simulink model "full_scale_car"  (R2024b)
settings: Solver=ode23t  StartTime=0.0  StopTime=25  MaxStep=1e-4  MinStep=1e-7  RelTol=1e-3
libraries: spsGroundLib x8, spsVoltageMeasurementLib x4, nesl_utility x4, spsControlledCurrentSourceLib x3, spsCurrentMeasurementLib x3, spsDCVoltageSourceLib x2, sdl_lib x2, spsSeriesRLCBranchLib x2, spsDCMachineLib x1, spsControlledVoltageSourceLib x1, fl_lib x1, simulink x1
settings Model: Creator=adamo  LastModifiedBy=adamo
settings SolverCC: ShapePreserveControl=EnableAll

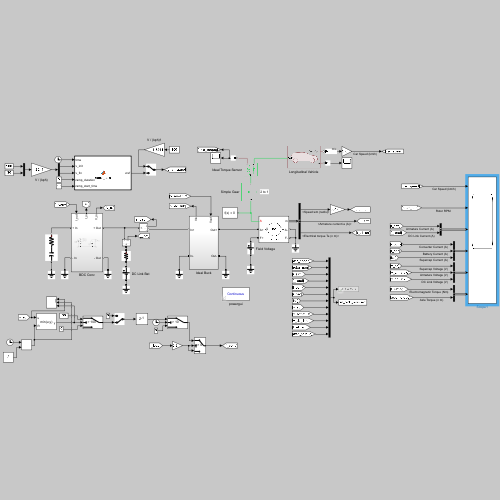
[thumbnail: Simulink's stored preview of the top-level diagram]
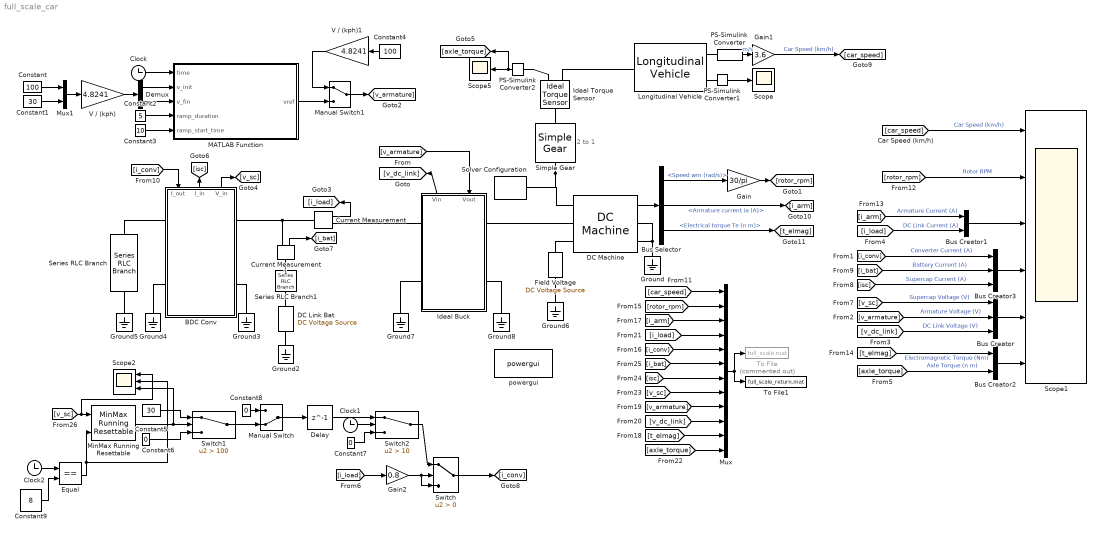
== system full_scale_car ==
  note: 2 to 1
  BDC Conv : Subsystem
      settings: PortSchema="{\"entries\":[{\"content\":{\"sides\":[{\"content\":{\"connectorIds\":[\"LConn1\",\"LConn2\"]},\"type\":\"ConnectorPlacement.EquallySpacedRectSide\",\"uuid\":\"9f090672-6a88-4e94-aaf3-d933b370ecea\"},{\"content\":{\"connectorIds\":[\"RConn1\",\"RConn2\"],\"side\":\"RIGHT\"},\"type\":\"ConnectorPlacement.EquallySpacedRectSide\",\"uuid\":\"4ec5d7b0-9e11-491f-a704-2c93c36a28cb\"},{\"content\":{\"connectorIds\":[\"In1\",\"Out1\",\"Out2\"],\"side\":\"TOP\"},\"type\":\"ConnectorPlacement.EquallySpacedRectSide\",\"uuid\":\"1397e6b8-a84b-4f43-abb0-36c2f8d57e37\"}]},\"type\":\"ConnectorPlacement.EquallySpacedConnector\",\"uuid\":\"02ba4b3a-9b7c-4d0b-ba36-63e783e5597b\"}],\"packageUris\":[\"http://schema.mathworks.com/mf0/Connector/R2020b\"],\"version\":\"1.0\"}"
  Bus Creator : BusCreator  Inputs=3
  Bus Creator1 : BusCreator  Inputs=2
  Bus Creator2 : BusCreator  Inputs=2
  Bus Creator3 : BusCreator  Inputs=3
  Bus Selector : BusSelector  OutputSignals=Speed wm (rad/s),Armature current ia (A),Electrical torque Te (n m)
  Clock : Clock
  Clock1 : Clock
  Clock2 : Clock
  Constant : Constant  Value=100
  Constant1 : Constant  Value=30
  Constant2 : Constant  Value=5
  Constant3 : Constant  Value=10
  Constant4 : Constant  Value=100
  Constant5 : Constant  Value=30
  Constant6 : Constant  Value=0
  Constant7 : Constant  Value=0
  Constant8 : Constant  Value=0
  Constant9 : Constant  Value=8
  Current Measurement : spsCurrentMeasurementLib/Current Measurement  PhasorSimulation=off  OutputType=Complex  PSBequivalent=0
  Current Measurement1 : spsCurrentMeasurementLib/Current Measurement  PhasorSimulation=off  OutputType=Complex  PSBequivalent=0
  DC Link Bat : spsDCVoltageSourceLib/DC Voltage Source  Amplitude=500  Measurements=None
  DC Machine : spsDCMachineLib/DC Machine  PresetModel=23: 250HP 500V 1750RPM Field:300V  MechanicalLoad=Mechanical rotational port  FieldType=Wound  ShowDetailedParameters=on  MeasurementBus=off  RLa=[0.06727 0.001882]  RLf=[30.72 3.166]  Laf=0.2641  MachineConstant=Torque constant (N.m/A)  Ke=1.8  Kt=1.8  J=1.019  Bm=0.02516  Tf=26.46  w0=190  Ifinit=9.76562499959051  TsPowergui=0  TsBlock=-1
  Delay : Delay  DelayLength=1
  Demux : Demux  Outputs=2
  Equal : RelationalOperator  Operator===  OutDataTypeStr=boolean  RndMeth=Simplest  InputSameDT=off
  Field Voltage : spsDCVoltageSourceLib/DC Voltage Source  Amplitude=300  Measurements=None
  Gain : Gain  Gain=30/pi
  Gain1 : Gain  Gain=3.6
  Gain2 : Gain  Gain=0.8
  Ground{,2..8} (8 alike) : spsGroundLib/Ground  LConnTagsString=a
  Ideal Buck : Subsystem
      settings: PortSchema="{\"entries\":[{\"content\":{\"sides\":[{\"content\":{\"connectorIds\":[\"LConn1\",\"LConn2\"]},\"type\":\"ConnectorPlacement.EquallySpacedRectSide\",\"uuid\":\"35f6ef1c-d887-4ecf-80f2-2c39dcd17f78\"},{\"content\":{\"connectorIds\":[\"RConn1\",\"RConn2\"],\"side\":\"RIGHT\"},\"type\":\"ConnectorPlacement.EquallySpacedRectSide\",\"uuid\":\"8a3f3d43-a013-4f94-8838-6f4ac1397b41\"},{\"content\":{\"connectorIds\":[\"Out1\",\"In1\"],\"side\":\"TOP\"},\"type\":\"ConnectorPlacement.EquallySpacedRectSide\",\"uuid\":\"6e5b1b24-962b-4715-9a1c-61b4175c500b\"}]},\"type\":\"ConnectorPlacement.EquallySpacedConnector\",\"uuid\":\"9f7927fc-518e-4b31-bc3b-cadb6b312eb4\"}],\"packageUris\":[\"http://schema.mathworks.com/mf0/Connector/R2020b\"],\"version\":\"1.0\"}"
  Ideal Torque Sensor : fl_lib/Mechanical/Mechanical Sensors/Ideal Torque Sensor
  Longitudinal Vehicle : sdl_lib/Tires & Vehicles/Longitudinal Vehicle  vehParamType=sdl.enum.VehicleParameterizationType.Regular  M_vehicle=2000 kg  R_tireroll=0.3 m  C_tireroll=0.0136  C_airdrag=0.4  A_front=2.3 m^2  A_rl=120 N  B_rl=1.8 N*s/m  C_rl=0.389 N*s^2/m^2  g=9.81 m/s^2  V_1=0.3 m/s  w_1=0.01 rad/s  ShowBrakeIn=false  ShowSlopeIn=false  SlopeInputType=sdl.enum.VehicleLongitudinalRoadSlopeInputType.GradePercent  ShowWindIn=false  ShowGOut=true  air_density=1.184 kg/m^3  V_x_specify=on  V_x_priority=High  V_x=100 kph  V_x_nominal_specify=on  V_x_nominal_value=100  V_x_nominal_unit=kph  trq_specify=off  trq_priority=None  trq=0 N*m  trq_nominal_specify=on  trq_nominal_value=150  trq_nominal_unit=N*m  w_specify=off  w_priority=None  w=0 rad/s  w_nominal_specify=on  w_nominal_value=190/3  w_nominal_unit=rad/s
      settings: InternalSimscapePortConfiguration="{\"Bottom\":[],\"Left\":[{\"id\":\"Axle\",\"label\":\"Axle\",\"type\":\"foundation.mechanical.rotational.rotational\"}],\"Right\":[{\"id\":\"v_out\",\"label\":\"VehSpd\",\"type\":\"output\"},{\"id\":\"G_out\",\"label\":\"G\",\"type\":\"output\"}],\"Top\":[]}"
  MATLAB Function : MATLAB Function  TreatAsAtomicUnit=on
  Manual Switch : ManualSwitch  CurrentSetting=0
  Manual Switch1 : ManualSwitch
  MinMax Running Resettable : simulink/Math Operations/MinMax Running Resettable  Function=min  vinit=200
  Mux : Mux  Inputs=12
  Mux1 : Mux  Inputs=2
  PS-Simulink Converter : nesl_utility/PS-Simulink Converter  PhysicalDomain=network_engine_domain  SubClassName=ps_output  LeftPortType=input  RightPortType=output  PseudoPeriodic=off  Frequencies=[]  VectorFormat=inherit  Unit=inherit  AffineConversion=off
  PS-Simulink Converter1 : nesl_utility/PS-Simulink Converter  PhysicalDomain=network_engine_domain  SubClassName=ps_output  LeftPortType=input  RightPortType=output  PseudoPeriodic=off  Frequencies=[]  VectorFormat=inherit  Unit=inherit  AffineConversion=off
  PS-Simulink Converter2 : nesl_utility/PS-Simulink Converter  PhysicalDomain=network_engine_domain  SubClassName=ps_output  LeftPortType=input  RightPortType=output  PseudoPeriodic=off  Frequencies=[]  VectorFormat=inherit  Unit=inherit  AffineConversion=off
  Scope : Scope
  Scope1 : Scope  NumInputPorts=6
  Scope2 : Scope  NumInputPorts=3
  Scope5 : Scope
  Series RLC Branch : spsSeriesRLCBranchLib/Series RLC Branch  LConnTagsString=__new0  RConnTagsString=__new0  BranchType=RC  Resistance=10e-3  Inductance=1e-3  SetiL0=off  InitialCurrent=0  Capacitance=20  Setx0=on  InitialVoltage=150  Measurements=None
  Series RLC Branch1 : spsSeriesRLCBranchLib/Series RLC Branch  LConnTagsString=__new0  RConnTagsString=__new0  BranchType=R  Resistance=10e-3  Inductance=1e-3  SetiL0=off  InitialCurrent=0  Capacitance=10  Setx0=on  InitialVoltage=250/4  Measurements=None
  Simple Gear : sdl_lib/Gears/Simple Gear  ratio=2  rotation_direction=sdl.enum.shaftOutputDirection.same  friction_model=sdl.enum.gear_efficiencies_load.off  T_noload=0.1 N*m  T_nom=5 N*m  efficiency_nom=0.8  efficiency=0.8  temperature_TLU=[280, 300, 320] K  load_TLU=[1, 5, 10] N*m  efficiency_TLU=[.95, .9, .85]  efficiency_TLU2=[.85, .8, .75; .95, .9, .85; .85, .8, .7]  w_thr=0.01 rad/s  pwr_thr=0.001 W  enable_backlash=false  hardstop_model=simscape.enum.hardstop.smooth  backlash_distance=1e-3 mm  r_base=0.1 m  transition=1e-4 mm  backlash_stiffness=1e6 N/m  backlash_damping=1e3 N*s/m  coeff_rest=0.7  v_tol=0.001 m/s  f_tol=0.001 N  mu_visc=[0, 0] N*m*s/rad  thermal_mass=50 J/K  temperature_specify=off  temperature_priority=High  temperature=300 K  temperature_nominal_specify=off  temperature_nominal_value=1  temperature_nominal_unit=K  x_backlash_specify=off  x_backlash_priority=None  x_backlash=0 mm  x_backlash_nominal_specify=off  x_backlash_nominal_value=1  x_backlash_nominal_unit=mm  f_hardstop_specify=off  f_hardstop_priority=None  f_hardstop=0 N  f_hardstop_nominal_specify=off  f_hardstop_nominal_value=1  f_hardstop_nominal_unit=N  v_backlash_specify=off  v_backlash_priority=None  v_backlash=0 m/s  v_backlash_nominal_specify=off  v_backlash_nominal_value=1  v_backlash_nominal_unit=m/s
  Solver Configuration : nesl_utility/Solver Configuration  PhysicalDomain=network_engine_domain  SubClassName=solver  LeftPortType=input  RightPortType=generic  Tones=[]  Harmonics=[]  SimulateNoise=off  Profile=off  UseLocalSampling=off  EnableSwitchedLinearOptims=on  FrequencyDomain=off  UseCCode=off  RelTol=0.001  AbsTol=0.001  MinStep=1e-09  ToWorkspace=off  RevertToSquareIcSolve=off  NumHomotopyIterations=100  PhasorMode=off  PhasorModeNumHarmonics=1  ConsistencySolver=NEWTON_XTOL_AFTER_FTOL  IndexReductionMethod=DerivativeReplacement  DoDC=off  ResidualTolerance=1e-09  ConsistencyTolSource=GLOBAL  ConsistencyAbsTol=0.001  ConsistencyRelTol=0.001  ConsistencyTolFactor=0.001  UseLocalSolver=off  LocalSolverChoice=NE_BACKWARD_EULER_ADVANCER  ResolveIndetEquations=on  FunctionEvalNumThread=1  LocalSolverSampleTime=0.001  DoFixedCost=off  MaxNonlinIter=3  MaxModeIter=2  ComputeImpulses=off  ImpulseIterations=2  LinearAlgebra=auto  LinearAlgebraNumThread=0  EquationFormulation=NE_TIME_EF  DelaysMemoryBudget=1024  AutomaticFiltering=on  FilteringTimeConstant=0.001  PartitionStorageMethod=AS_NEEDED  PartitionMemoryBudget=1024  PartitionMethod=ROBUST  MultibodyUseLocalSolver=off  MultibodyLocalSolverChoice=ODE1  MultibodyLocalSolverSampleTime=0.001
  Switch : Switch  Criteria=u2 > Threshold  SaturateOnIntegerOverflow=off  InputSameDT=off
  Switch1 : Switch  Criteria=u2 > Threshold  Threshold=100  SaturateOnIntegerOverflow=off  InputSameDT=off
  Switch2 : Switch  Criteria=u2 > Threshold  Threshold=10  SaturateOnIntegerOverflow=off  InputSameDT=off
  To File : ToFile  Commented=on  Filename=full_scale.mat  MatrixName=fs_ans
  To File1 : ToFile  Filename=full_scale_return.mat  MatrixName=fs_ans
  V / (kph) : Gain  Gain=4.8241
  V / (kph)1 : Gain  Gain=4.8241
  powergui : spspowerguiLib/powergui  Priority=1  SimulationMode=Continuous  SampleTime=50e-6  frequency=60  Iterations=50  frequencyindice=0  Pbase=100e6  ErrMax=1e-4  UnitsV=kV  UnitsW=MW  buscounter=0  FunctionMessages=off  echomessages=off  EnableUseOfTLC=off  CurrentSourceSwitches=off  DisableSnubberDevices=on  DisableRonSwitches=on  DisableVfSwitches=on  DisplayEquations=off  AutomaticDiscreteSolvers=off  SolverType=Tustin/Backward Euler (TBE)  Interpol=off  ExternalGateDelay=off  methode=off  Ts=100  x0status=blocks  SPID=on  SwTol=0  HookPort=off  NonlinearTolerance=1e-4  nMaxIteration=100  ContinueOnMaxIteration=off  RestoreLinks=warning  ResistiveCurrentMeasurement=off  Frange=[0:2:500]  Ylog=off  Xlog=on  ShowGrid=off  save=off  variable=ZData  structure=0  ZoomFFT=off  StartTime=0.0  cycles=1  DisplayStyle=1  fundamental=60  FreqAxis=off  MaxFrequency=1000  frequencyindicesteady=1  RmsSteady=1  display=off
  wires:
  [axle_torque] -> Bus Creator2/2  "Axle Torque (n m)"
  Gain1/1 -> [car_speed]  "Car Speed (km/h)"
  Bus Selector/2 -> [i_arm]  "<Armature current ia (A)>"
  Bus Creator/1 -> Scope1/5
  Bus Selector/1 -> Gain/1  "<Speed wm (rad/s)>"
  Gain/1 -> [rotor_rpm]
  [t_elmag] -> Bus Creator2/1  "Electromagnetic Torque (Nm)"
  Bus Creator2/1 -> Scope1/6
  Bus Creator1/1 -> Scope1/3
  DC Machine/1 -> Bus Selector/1
  [i_load] -> Bus Creator1/2  "DC Link Current (A)"
  PS-Simulink Converter2/1 -> [axle_torque], Scope5/1
  PS-Simulink Converter/1 -> Gain1/1  "m/s"
  [v_armature] -> Bus Creator/2  "Armature Voltage (V)"
  [v_dc_link] -> Bus Creator/3  "DC Link Voltage (V)"
  Current Measurement/1 -> [i_load]
  MATLAB Function/1(vref) -> Manual Switch1/2
  [v_armature] -> Ideal Buck/1(Vout)
  Ideal Buck/1(Vin) -> [v_dc_link]
  Clock/1 -> MATLAB Function/1(time)
  Constant2/1 -> MATLAB Function/4(ramp_duration)
  Constant3/1 -> MATLAB Function/5(ramp_start_time)
  [v_sc] -> Bus Creator/1  "Supercap Voltage (V)"
  [isc] -> Bus Creator3/3  "Supercap Current (A)"
  Current Measurement1/1 -> [i_bat]
  [i_bat] -> Bus Creator3/2  "Battery Current (A)"
  BDC Conv/1(I_in) -> [isc]
  Bus Creator3/1 -> Scope1/4
  [i_conv] -> Bus Creator3/1  "Converter Current (A)"
  PS-Simulink Converter1/1 -> Scope/1
  BDC Conv/2(V_in) -> [v_sc]
  [i_conv] -> BDC Conv/1(I_out)
  [i_load] -> Gain2/1
  Manual Switch/1 -> Delay/1
  Gain2/1 -> Switch/2, Switch/3
  [car_speed] -> Scope1/1  "Car Speed (km/h)"
  [rotor_rpm] -> Scope1/2  "Rotor RPM"
  [i_arm] -> Bus Creator1/1  "Armature Current (A)"
  Bus Selector/3 -> [t_elmag]  "<Electrical torque Te (n m)>"
  [axle_torque] -> Mux/12
  [car_speed] -> Mux/1
  [rotor_rpm] -> Mux/2
  [i_arm] -> Mux/3
  [i_load] -> Mux/4
  [i_conv] -> Mux/5
  [i_bat] -> Mux/6
  [isc] -> Mux/7
  [v_sc] -> Mux/8
  [v_armature] -> Mux/9
  [v_dc_link] -> Mux/10
  [t_elmag] -> Mux/11
  Mux/1 -> To File/1, To File1/1
  Constant1/1 -> Mux1/2
  Constant/1 -> Mux1/1
  V / (kph)/1 -> Demux/1
  Demux/1 -> MATLAB Function/2(v_init)
  Demux/2 -> MATLAB Function/3(v_fin)
  Mux1/1 -> V / (kph)/1
  Switch1/1 -> Manual Switch/2
  Constant5/1 -> Switch1/1
  Constant6/1 -> Switch1/3
  Constant8/1 -> Manual Switch/1
  Switch/1 -> [i_conv]
  Constant4/1 -> V / (kph)1/1
  V / (kph)1/1 -> Manual Switch1/1
  Manual Switch1/1 -> [v_armature]
  Switch2/1 -> Switch/1
  Delay/1 -> Switch2/1
  Clock1/1 -> Switch2/2
  Constant7/1 -> Switch2/3
  MinMax Running Resettable/1 -> Scope2/3, Switch1/2
  [v_sc] -> Scope2/1, MinMax Running Resettable/1
  Clock2/1 -> Equal/1
  Constant9/1 -> Equal/2
  Equal/1 -> MinMax Running Resettable/2, Scope2/2
  connections:
  Simple Gear/LConn1 -- DC Machine/LConn1 -- Solver Configuration/RConn1
  Current Measurement/RConn1 -- Ideal Buck/LConn1
  Field Voltage/RConn1 -- DC Machine/LConn3
  Longitudinal Vehicle/RConn1 -- PS-Simulink Converter/LConn1
  PS-Simulink Converter2/LConn1 -- Ideal Torque Sensor/RConn2
  PS-Simulink Converter1/LConn1 -- Longitudinal Vehicle/RConn2
  Ideal Torque Sensor/RConn1 -- Longitudinal Vehicle/LConn1
  Ideal Torque Sensor/LConn1 -- Simple Gear/RConn1
  Ground/LConn1 -- DC Machine/RConn2 -- DC Machine/RConn1
  Ground3/LConn1 -- BDC Conv/RConn2
  Current Measurement/LConn1 -- Current Measurement1/RConn1 -- BDC Conv/RConn1
  BDC Conv/LConn2 -- Ground4/LConn1
  Series RLC Branch/RConn1 -- Ground5/LConn1
  Ground6/LConn1 -- Field Voltage/LConn1
  Ideal Buck/LConn2 -- Ground7/LConn1
  Ground8/LConn1 -- Ideal Buck/RConn2
  BDC Conv/LConn1 -- Series RLC Branch/LConn1
  Series RLC Branch1/LConn1 -- Current Measurement1/LConn1
  Series RLC Branch1/RConn1 -- DC Link Bat/RConn1
  Ground2/LConn1 -- DC Link Bat/LConn1
  DC Machine/LConn2 -- Ideal Buck/RConn1

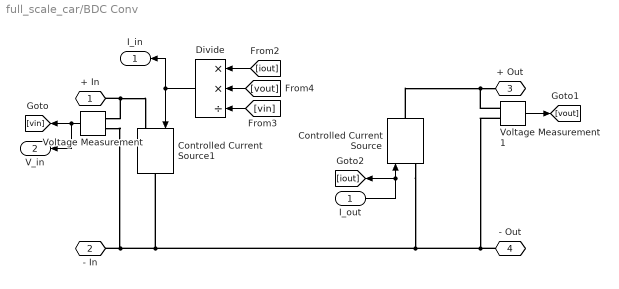
== system full_scale_car/BDC Conv ==
  I_out : Inport
  Controlled Current Source : spsControlledCurrentSourceLib/Controlled Current Source  Initialize=on  Source_Type=DC  Amplitude=0  Phase=0  Frequency=0  Measurements=None
  Controlled Current Source1 : spsControlledCurrentSourceLib/Controlled Current Source  Initialize=on  Source_Type=DC  Amplitude=0  Phase=0  Frequency=0  Measurements=None
  Divide : Product  Inputs=**/
  Voltage Measurement : spsVoltageMeasurementLib/Voltage Measurement  PhasorSimulation=off  OutputType=Complex  PSBequivalent=0
  Voltage Measurement1 : spsVoltageMeasurementLib/Voltage Measurement  PhasorSimulation=off  OutputType=Complex  PSBequivalent=0
  + In : PMIOPort  Side=Left
  - In : PMIOPort  Port=2  Side=Left
  "+ Out " : PMIOPort  Port=3  Side=Right
  "- Out " : PMIOPort  Port=4  Side=Right
  I_in : Outport
  V_in : Outport  Port=2
  wires:
  Voltage Measurement/1 -> V_in/1, [vin]
  Voltage Measurement1/1 -> [vout]
  [vin] -> Divide/3
  [vout] -> Divide/2
  [iout] -> Divide/1
  I_out/1 -> [iout], Controlled Current Source/1
  Divide/1 -> Controlled Current Source1/1, I_in/1
  connections:
  Controlled Current Source/RConn1 -- Voltage Measurement1/LConn1 -- "+ Out "/RConn1
  "- Out "/RConn1 -- Voltage Measurement1/LConn2 -- Controlled Current Source/LConn1 -- Voltage Measurement/LConn2 -- - In/RConn1 -- Controlled Current Source1/RConn1
  Voltage Measurement/LConn1 -- Controlled Current Source1/LConn1 -- + In/RConn1

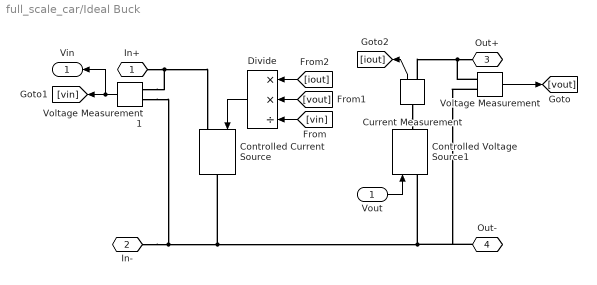
== system full_scale_car/Ideal Buck ==
  Vout : Inport
  Controlled Current Source : spsControlledCurrentSourceLib/Controlled Current Source  Initialize=on  Source_Type=DC  Amplitude=5  Phase=0  Frequency=0  Measurements=None
  Controlled Voltage Source1 : spsControlledVoltageSourceLib/Controlled Voltage Source  Initialize=on  Source_Type=DC  Amplitude=250  Phase=0  Frequency=0  Measurements=None
  Current Measurement : spsCurrentMeasurementLib/Current Measurement  PhasorSimulation=off  OutputType=Complex  PSBequivalent=0
  Divide : Product  Inputs=**/
  Voltage Measurement : spsVoltageMeasurementLib/Voltage Measurement  PhasorSimulation=off  OutputType=Complex  PSBequivalent=0
  Voltage Measurement1 : spsVoltageMeasurementLib/Voltage Measurement  PhasorSimulation=off  OutputType=Complex  PSBequivalent=0
  In+ : PMIOPort  Side=Left
  In- : PMIOPort  Port=2  Side=Left
  Out+ : PMIOPort  Port=3  Side=Right
  Out- : PMIOPort  Port=4  Side=Right
  Vin : Outport
  wires:
  Vout/1 -> Controlled Voltage Source1/1
  Voltage Measurement1/1 -> Vin/1, [vin]
  Voltage Measurement/1 -> [vout]
  Current Measurement/1 -> [iout]
  Divide/1 -> Controlled Current Source/1
  [vin] -> Divide/3
  [iout] -> Divide/1
  [vout] -> Divide/2
  connections:
  In-/RConn1 -- Voltage Measurement1/LConn2 -- Voltage Measurement/LConn2 -- Out-/RConn1 -- Controlled Voltage Source1/LConn1 -- Controlled Current Source/RConn1
  In+/RConn1 -- Voltage Measurement1/LConn1 -- Controlled Current Source/LConn1
  Voltage Measurement/LConn1 -- Current Measurement/RConn1 -- Out+/RConn1
  Current Measurement/LConn1 -- Controlled Voltage Source1/RConn1

== matlab function full_scale_car/MATLAB Function ==
  data: time input; vref output; v_init input; v_fin input; ramp_duration input; ramp_start_time input
function vref = ramp_calc(time,v_init,v_fin, ramp_duration, ramp_start_time)
    
    slope=(v_fin - v_init) / ramp_duration;
    if time<=ramp_start_time
        vref=v_init;
    else
        if time>(ramp_start_time+ramp_duration)
        vref=v_fin;
        else
            vref=v_init+slope*(time-ramp_start_time);
        end
    end
